simulink model "Res_21"  (R2018b)
settings: Solver=ode4  StartTime=0.0  StopTime=0.5  RelTol=1e-3
values from neighbouring files (symbols this model uses):
  A = [0 1 0 0;-k/j1 -b/j1 k/j2 0;0 0 0 1;k/j2 0 -k/j2 -b/j2]    [result_21.m]
  B = [0;-1/j1;0;1/j2]    [result_21.m]
  C = [-1 0 1 0]    [result_21.m]
  D = [0]    [result_21.m]
settings Model: Creator=makha  LastModifiedBy=makha

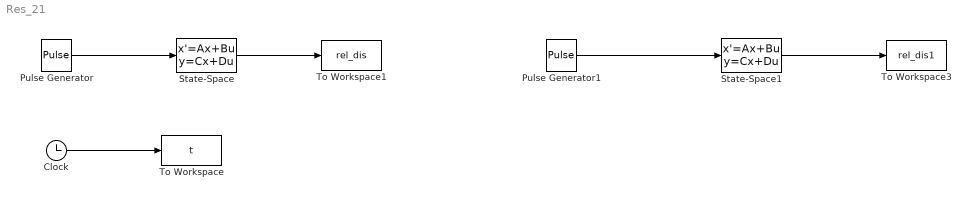
== system Res_21 ==
  Clock : Clock
  Pulse Generator : DiscretePulseGenerator  PulseType=Time based  Amplitude=5500  Period=0.02  PulseWidth=10  PhaseDelay=0.0001
  Pulse Generator1 : DiscretePulseGenerator  PulseType=Time based  Amplitude=5500  Period=0.0314  PulseWidth=10  PhaseDelay=0.0001
  State-Space : StateSpace  A=A  B=B  C=C  D=D  InitialCondition=zeros(4,1)
  State-Space1 : StateSpace  A=A  B=B  C=C  D=D  InitialCondition=zeros(4,1)
  To Workspace : ToWorkspace  VariableName=t  SampleTime=-1
  To Workspace1 : ToWorkspace  VariableName=rel_dis  SampleTime=-1
  To Workspace3 : ToWorkspace  VariableName=rel_dis1  SampleTime=-1
  wires:
  Pulse Generator/1 -> State-Space/1
  State-Space/1 -> To Workspace1/1
  Clock/1 -> To Workspace/1
  Pulse Generator1/1 -> State-Space1/1
  State-Space1/1 -> To Workspace3/1
